simulink model "Model_P1"  (R2022b)
settings: Solver=FixedStepAuto  StartTime=0.0  StopTime=10000  FixedStep=1  RelTol=1e-3
undefined symbols (not defined in the file): current_hyst, gamma_, hyst_M, OCV, R0, SOC_levels
settings Model: Creator=frederikvanmaele  LastModifiedBy=AdministratorDevice
settings DebuggingCC: UnconnectedInputMsg=warning  UnconnectedOutputMsg=warning  UnconnectedLineMsg=warning
settings ModelReferenceCC: EnableRefExpFcnMdlSchedulingChecks=on
settings RTWCC: DLArmComputeVersion=19.05

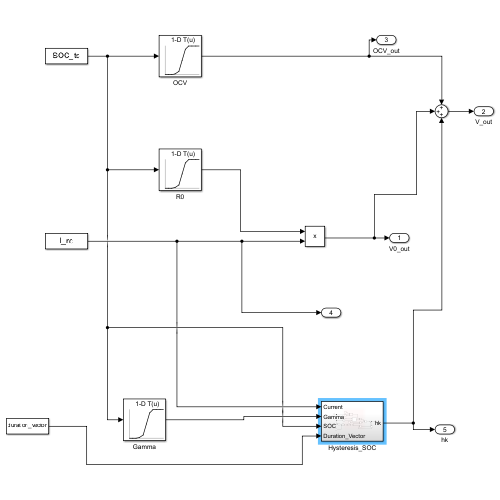
[thumbnail: Simulink's stored preview of the top-level diagram]
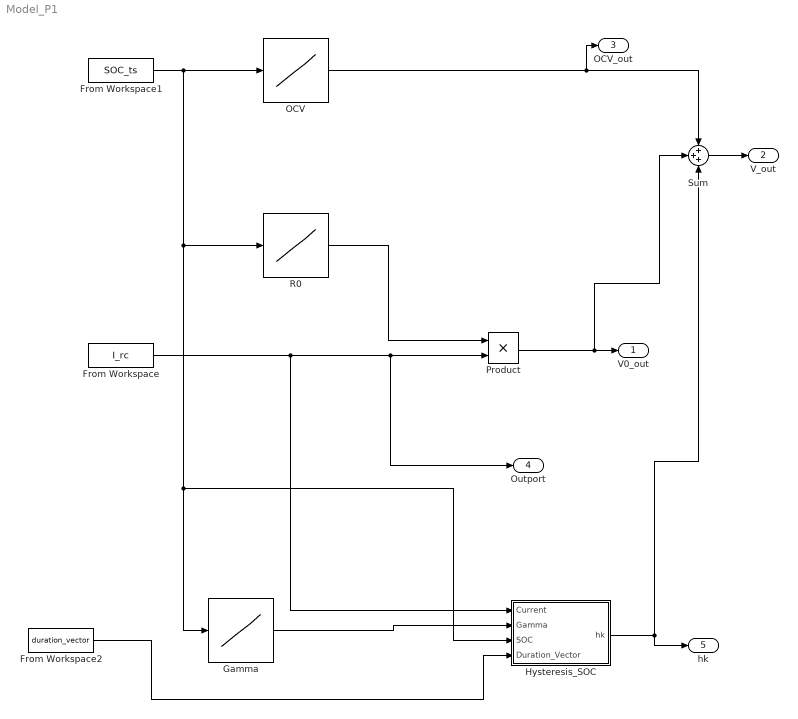
== system Model_P1 ==
  From Workspace : FromWorkspace  VariableName=I_rc
  From Workspace1 : FromWorkspace  VariableName=SOC_ts
  From Workspace2 : FromWorkspace  VariableName=duration_vector
  Gamma : Lookup_n-D  NumberOfTableDimensions=1  BreakpointsForDimension1=SOC_levels  Table=gamma_  InternalRulePriority=Speed  RndMeth=Simplest
  Hysteresis_SOC : Subsystem
  OCV : Lookup_n-D  NumberOfTableDimensions=1  BreakpointsForDimension1=SOC_levels  Table=OCV  InternalRulePriority=Speed  RndMeth=Simplest
  Product : Product
  R0 : Lookup_n-D  NumberOfTableDimensions=1  BreakpointsForDimension1=SOC_levels  Table=R0  InternalRulePriority=Speed  RndMeth=Simplest
  Sum : Sum  Inputs=+++
  V0_out : Outport
  V_out : Outport  Port=2
  OCV_out : Outport  Port=3
  Outport : Outport  Port=4
  hk : Outport  Port=5
  wires:
  Product/1 -> Sum/2, V0_out/1
  From Workspace/1 -> Outport/1, Product/2, Hysteresis_SOC/1(Current)
  Sum/1 -> V_out/1
  Gamma/1 -> Hysteresis_SOC/2(Gamma)
  Hysteresis_SOC/1(hk) -> Sum/3, hk/1
  OCV/1 -> Sum/1, OCV_out/1
  R0/1 -> Product/1
  From Workspace1/1 -> Hysteresis_SOC/3(SOC), Gamma/1, R0/1, OCV/1
  From Workspace2/1 -> Hysteresis_SOC/4(Duration_Vector)

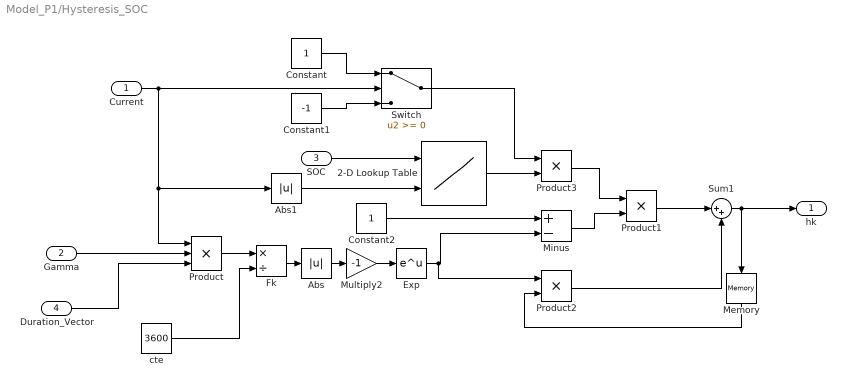
== system Model_P1/Hysteresis_SOC ==
  Current : Inport
  Gamma : Inport  Port=2
  SOC : Inport  Port=3
  Duration_Vector : Inport  Port=4
  2-D Lookup Table : Lookup_n-D  BreakpointsForDimension1=SOC_levels  BreakpointsForDimension2=current_hyst  Table=hyst_M  ExtrapMethod=Clip  UseLastTableValue=on  InternalRulePriority=Speed  RndMeth=Simplest
      settings: InputPortMap=u0,u1
  Abs : Abs  SaturateOnIntegerOverflow=off
  Abs1 : Abs  SaturateOnIntegerOverflow=off
  Constant : Constant
  Constant1 : Constant  Value=-1
  Constant2 : Constant
  Exp : Math
  Fk : Product  Inputs=*/
  Memory : Memory
  Minus : Sum  Inputs=+-
  Multiply2 : Gain  Gain=-1
  Product : Product  Inputs=3
  Product1 : Product
  Product2 : Product
  Product3 : Product
  Sum1 : Sum  Inputs=|++
  Switch : Switch  SaturateOnIntegerOverflow=off  InputSameDT=off
  cte : Constant  Value=3600
  hk : Outport
  wires:
  Product2/1 -> Sum1/2
  Memory/1 -> Product2/2
  Minus/1 -> Product1/2
  Product1/1 -> Sum1/1
  cte/1 -> Fk/2
  Gamma/1 -> Product/2
  Product/1 -> Fk/1
  Constant2/1 -> Minus/1
  Exp/1 -> Product2/1, Minus/2
  Current/1 -> Switch/2, Product/1, Abs1/1
  2-D Lookup Table/1 -> Product3/2
  Sum1/1 -> hk/1, Memory/1
  Duration_Vector/1 -> Product/3
  Constant/1 -> Switch/1
  Constant1/1 -> Switch/3
  Switch/1 -> Product3/1
  Product3/1 -> Product1/1
  Multiply2/1 -> Exp/1
  Fk/1 -> Abs/1
  Abs/1 -> Multiply2/1
  SOC/1 -> 2-D Lookup Table/1
  Abs1/1 -> 2-D Lookup Table/2
